simulink model "wbs_sim"  (R2025a)
settings: Solver=FixedStepAuto  StartTime=0.0  StopTime=20  FixedStep=0.001  RelTol=1e-3
undefined symbols (not defined in the file or in its folder): dyaw, L_l, L_r, phi_1l, phi_1r, phi_4l, phi_4r, roll, theta_l, theta_r, x, X, Y, yaw, Z
libraries: sm_lib x86, nesl_utility x28, slpidlib x6
(part 4 of 4)

== system wbs_sim/simscape model/物理系统/左腿/大腿后 ==
  Rigid Transform1 : sm_lib/Frames and Transforms/Rigid Transform  RotationMethod=None  FollAlignAxisA=+X  BaseAlignAxisA=+Y  FollAlignAxisB=+Y  BaseAlignAxisB=+Z  RotationStandardAxis=+Z  RotationAngle=0.0  RotationAngleUnits=deg  RotationArbitraryAxis=[0 0 1]  RotationSequenceAxes=FollowerAxes  RotationSequence=XYX  RotationSequenceAngles=[0 0 0]  RotationSequenceAnglesUnits=deg  RotationMatrix=[1 0 0; 0 1 0; 0 0 1]  Quaternion=[1 0 0 0]  TranslationMethod=StandardAxis  TranslationCartesianOffset=[0 0 0]  TranslationCartesianOffsetUnits=m  TranslationStandardAxis=+X  TranslationStandardOffset=L/2  TranslationStandardOffsetUnits=m  TranslationROffset=0  TranslationROffsetUnits=m  TranslationThetaOffset=0  TranslationThetaOffsetUnits=deg  TranslationZOffset=0  TranslationZOffsetUnits=m
  Rigid Transform3 : sm_lib/Frames and Transforms/Rigid Transform  RotationMethod=None  FollAlignAxisA=+X  BaseAlignAxisA=+Y  FollAlignAxisB=+Y  BaseAlignAxisB=+Z  RotationStandardAxis=+Z  RotationAngle=0.0  RotationAngleUnits=deg  RotationArbitraryAxis=[0 0 1]  RotationSequenceAxes=FollowerAxes  RotationSequence=XYX  RotationSequenceAngles=[0 0 0]  RotationSequenceAnglesUnits=deg  RotationMatrix=[1 0 0; 0 1 0; 0 0 1]  Quaternion=[1 0 0 0]  TranslationMethod=StandardAxis  TranslationCartesianOffset=[0 0 0]  TranslationCartesianOffsetUnits=m  TranslationStandardAxis=+X  TranslationStandardOffset=L/2  TranslationStandardOffsetUnits=m  TranslationROffset=0  TranslationROffsetUnits=m  TranslationThetaOffset=0  TranslationThetaOffsetUnits=deg  TranslationZOffset=0  TranslationZOffsetUnits=m
  Solid : sm_lib/Body Elements/Brick Solid  BrickDimensions=[L H W]  BrickDimensionsUnits=m  ExportEntireGeometry=off  InertiaType=CalculateFromGeometry  BasedOnType=Mass  Density=Mass  DensityUnits=kg/m^3  Mass=mass  MassUnits=kg  CenterOfMass=[0 0 0]  CenterOfMassUnits=m  MomentsOfInertia=[1 1 1]  MomentsOfInertiaUnits=kg*m^2  ProductsOfInertia=[0 0 0]  ProductsOfInertiaUnits=kg*m^2  GraphicType=FromGeometry  MarkerShape=Sphere  MarkerSize=10  GraphicVisPropType=SimpleVisualProperties  GraphicDiffuseColor=[0.6667 0 1]  GraphicOpacity=1.0  GraphicSpecularColor=[0.5 0.5 0.5 1.0]  GraphicAmbientColor=[0.15 0.15 0.15 1.0]  GraphicEmissiveColor=[0.0 0.0 0.0 1.0]  GraphicShininess=75  DoExposeReferenceFrame=on  SerializedFrames=<Frames/>
  Conn1 : PMIOPort  Side=Left
  Conn2 : PMIOPort  Port=2  Side=Right
  connections:
  Solid/RConn1 -- Rigid Transform3/RConn1 -- Rigid Transform1/LConn1
  Conn1/RConn1 -- Rigid Transform3/LConn1
  Rigid Transform1/RConn1 -- Conn2/RConn1

== system wbs_sim/simscape model/物理系统/左腿/小腿前 ==
  Rigid Transform1 : sm_lib/Frames and Transforms/Rigid Transform  RotationMethod=None  FollAlignAxisA=+X  BaseAlignAxisA=+Y  FollAlignAxisB=+Y  BaseAlignAxisB=+Z  RotationStandardAxis=+Z  RotationAngle=0.0  RotationAngleUnits=deg  RotationArbitraryAxis=[0 0 1]  RotationSequenceAxes=FollowerAxes  RotationSequence=XYX  RotationSequenceAngles=[0 0 0]  RotationSequenceAnglesUnits=deg  RotationMatrix=[1 0 0; 0 1 0; 0 0 1]  Quaternion=[1 0 0 0]  TranslationMethod=StandardAxis  TranslationCartesianOffset=[0 0 0]  TranslationCartesianOffsetUnits=m  TranslationStandardAxis=+X  TranslationStandardOffset=L/2  TranslationStandardOffsetUnits=m  TranslationROffset=0  TranslationROffsetUnits=m  TranslationThetaOffset=0  TranslationThetaOffsetUnits=deg  TranslationZOffset=0  TranslationZOffsetUnits=m
  Rigid Transform3 : sm_lib/Frames and Transforms/Rigid Transform  RotationMethod=None  FollAlignAxisA=+X  BaseAlignAxisA=+Y  FollAlignAxisB=+Y  BaseAlignAxisB=+Z  RotationStandardAxis=+Z  RotationAngle=0.0  RotationAngleUnits=deg  RotationArbitraryAxis=[0 0 1]  RotationSequenceAxes=FollowerAxes  RotationSequence=XYX  RotationSequenceAngles=[0 0 0]  RotationSequenceAnglesUnits=deg  RotationMatrix=[1 0 0; 0 1 0; 0 0 1]  Quaternion=[1 0 0 0]  TranslationMethod=StandardAxis  TranslationCartesianOffset=[0 0 0]  TranslationCartesianOffsetUnits=m  TranslationStandardAxis=+X  TranslationStandardOffset=L/2  TranslationStandardOffsetUnits=m  TranslationROffset=0  TranslationROffsetUnits=m  TranslationThetaOffset=0  TranslationThetaOffsetUnits=deg  TranslationZOffset=0  TranslationZOffsetUnits=m
  Solid : sm_lib/Body Elements/Brick Solid  BrickDimensions=[L H W]  BrickDimensionsUnits=m  ExportEntireGeometry=off  InertiaType=CalculateFromGeometry  BasedOnType=Mass  Density=mass  DensityUnits=kg/m^3  Mass=mass  MassUnits=kg  CenterOfMass=[0 0 0]  CenterOfMassUnits=m  MomentsOfInertia=[1 1 1]  MomentsOfInertiaUnits=kg*m^2  ProductsOfInertia=[0 0 0]  ProductsOfInertiaUnits=kg*m^2  GraphicType=FromGeometry  MarkerShape=Sphere  MarkerSize=10  GraphicVisPropType=SimpleVisualProperties  GraphicDiffuseColor=[1 0 1]  GraphicOpacity=1.0  GraphicSpecularColor=[0.5 0.5 0.5 1.0]  GraphicAmbientColor=[0.15 0.15 0.15 1.0]  GraphicEmissiveColor=[0.0 0.0 0.0 1.0]  GraphicShininess=75  DoExposeReferenceFrame=on  SerializedFrames=<Frames/>
  Conn1 : PMIOPort  Side=Left
  Conn2 : PMIOPort  Port=2  Side=Right
  connections:
  Rigid Transform1/RConn1 -- Conn2/RConn1
  Conn1/RConn1 -- Rigid Transform3/LConn1
  Rigid Transform1/LConn1 -- Solid/RConn1 -- Rigid Transform3/RConn1

== system wbs_sim/simscape model/物理系统/左腿/小腿后 ==
  Rigid Transform1 : sm_lib/Frames and Transforms/Rigid Transform  RotationMethod=None  FollAlignAxisA=+X  BaseAlignAxisA=+Y  FollAlignAxisB=+Y  BaseAlignAxisB=+Z  RotationStandardAxis=+Z  RotationAngle=0.0  RotationAngleUnits=deg  RotationArbitraryAxis=[0 0 1]  RotationSequenceAxes=FollowerAxes  RotationSequence=XYX  RotationSequenceAngles=[0 0 0]  RotationSequenceAnglesUnits=deg  RotationMatrix=[1 0 0; 0 1 0; 0 0 1]  Quaternion=[1 0 0 0]  TranslationMethod=StandardAxis  TranslationCartesianOffset=[0 0 0]  TranslationCartesianOffsetUnits=m  TranslationStandardAxis=+X  TranslationStandardOffset=L/2  TranslationStandardOffsetUnits=m  TranslationROffset=0  TranslationROffsetUnits=m  TranslationThetaOffset=0  TranslationThetaOffsetUnits=deg  TranslationZOffset=0  TranslationZOffsetUnits=m
  Rigid Transform3 : sm_lib/Frames and Transforms/Rigid Transform  RotationMethod=None  FollAlignAxisA=+X  BaseAlignAxisA=+Y  FollAlignAxisB=+Y  BaseAlignAxisB=+Z  RotationStandardAxis=+Z  RotationAngle=0.0  RotationAngleUnits=deg  RotationArbitraryAxis=[0 0 1]  RotationSequenceAxes=FollowerAxes  RotationSequence=XYX  RotationSequenceAngles=[0 0 0]  RotationSequenceAnglesUnits=deg  RotationMatrix=[1 0 0; 0 1 0; 0 0 1]  Quaternion=[1 0 0 0]  TranslationMethod=StandardAxis  TranslationCartesianOffset=[0 0 0]  TranslationCartesianOffsetUnits=m  TranslationStandardAxis=+X  TranslationStandardOffset=L/2  TranslationStandardOffsetUnits=m  TranslationROffset=0  TranslationROffsetUnits=m  TranslationThetaOffset=0  TranslationThetaOffsetUnits=deg  TranslationZOffset=0  TranslationZOffsetUnits=m
  Solid : sm_lib/Body Elements/Brick Solid  BrickDimensions=[L H W]  BrickDimensionsUnits=m  ExportEntireGeometry=off  InertiaType=CalculateFromGeometry  BasedOnType=Mass  Density=mass  DensityUnits=kg/m^3  Mass=mass  MassUnits=kg  CenterOfMass=[0 0 0]  CenterOfMassUnits=m  MomentsOfInertia=[1 1 1]  MomentsOfInertiaUnits=kg*m^2  ProductsOfInertia=[0 0 0]  ProductsOfInertiaUnits=kg*m^2  GraphicType=FromGeometry  MarkerShape=Sphere  MarkerSize=10  GraphicVisPropType=SimpleVisualProperties  GraphicDiffuseColor=[1 0 1]  GraphicOpacity=1.0  GraphicSpecularColor=[0.5 0.5 0.5 1.0]  GraphicAmbientColor=[0.15 0.15 0.15 1.0]  GraphicEmissiveColor=[0.0 0.0 0.0 1.0]  GraphicShininess=75  DoExposeReferenceFrame=on  SerializedFrames=<Frames/>
  Conn1 : PMIOPort  Side=Left
  Conn2 : PMIOPort  Port=2  Side=Right
  connections:
  Rigid Transform1/RConn1 -- Conn2/RConn1
  Conn1/RConn1 -- Rigid Transform3/LConn1
  Rigid Transform1/LConn1 -- Solid/RConn1 -- Rigid Transform3/RConn1

== matlab function wbs_sim/controller/left leg transform ==
  data: F input; Tp input; T output; phi1 input; phi4 input
function T = LegTransform(F,Tp,phi1,phi4)
%LegTransform
%    T = LegTransform(F,Tp,PHI1,PHI4)

%    This function was generated by the Symbolic Math Toolbox version 25.1.
%    2025-11-06 00:02:19

t2 = conj(phi1);
t3 = conj(phi4);
t4 = cos(phi1);
t5 = cos(phi4);
t6 = sin(phi1);
t7 = sin(phi4);
t8 = cos(t2);
t9 = cos(t3);
t10 = imag(t4);
t11 = real(t4);
t12 = sin(t2);
t13 = sin(t3);
t14 = imag(t6);
t15 = real(t6);
t16 = t4.*(2.1e+1./1.0e+2);
t17 = t5.*(2.1e+1./1.0e+2);
t18 = t4.*(2.1e+1./2.0e+2);
t19 = t5.*(2.1e+1./2.0e+2);
t20 = t6.*(2.1e+1./1.0e+2);
t21 = t7.*(2.1e+1./1.0e+2);
t22 = t6.*(2.1e+1./2.0e+2);
t23 = t7.*(2.1e+1./2.0e+2);
t24 = -t17;
t25 = -t18;
t26 = -t19;
t27 = -t21;
t28 = -t22;
t29 = -t23;
t30 = t8.*(2.1e+1./1.0e+2);
t31 = t9.*(2.1e+1./1.0e+2);
t32 = t8.*(2.1e+1./2.0e+2);
t33 = t9.*(2.1e+1./2.0e+2);
t34 = t10.*(2.1e+1./1.0e+2);
t35 = t11.*(2.1e+1./1.0e+2);
t36 = t12.*(2.1e+1./1.0e+2);
t37 = t13.*(2.1e+1./1.0e+2);
t38 = t12.*(2.1e+1./2.0e+2);
t39 = t13.*(2.1e+1./2.0e+2);
t40 = t14.*(2.1e+1./1.0e+2);
t41 = t15.*(2.1e+1./1.0e+2);
t42 = -t31;
t43 = -t32;
t44 = -t33;
t45 = -t37;
t46 = -t38;
t47 = -t39;
t48 = -t40;
t49 = t16+t24;
t50 = t18+t26;
t51 = t20+t27;
t52 = t22+t29;
t53 = t49.^2;
t54 = t50.^2;
t55 = t51.^2;
t56 = t52.^2;
t57 = t30+t42;
t58 = t32+t44;
t59 = t36+t45;
t60 = t38+t47;
t63 = t6.*t49.*(2.1e+1./5.0e+1);
t64 = t7.*t49.*(2.1e+1./5.0e+1);
t65 = t4.*t51.*(2.1e+1./5.0e+1);
t66 = t5.*t51.*(2.1e+1./5.0e+1);
t73 = t16.*t52;
t75 = t6.*t50.*(-2.1e+1./1.0e+2);
t76 = t7.*t50.*(-2.1e+1./1.0e+2);
t61 = t59.^2;
t62 = t57.^2;
t67 = -t63;
t68 = -t64;
t71 = -t65;
t72 = -t66;
t77 = t12.*t57.*(2.1e+1./5.0e+1);
t78 = t13.*t57.*(2.1e+1./5.0e+1);
t79 = t8.*t59.*(2.1e+1./5.0e+1);
t80 = t9.*t59.*(2.1e+1./5.0e+1);
t87 = t30.*t60;
t89 = t12.*t58.*(-2.1e+1./1.0e+2);
t90 = t13.*t58.*(-2.1e+1./1.0e+2);
t91 = t53+t55;
t81 = -t77;
t82 = -t78;
t85 = -t79;
t86 = -t80;
t92 = t91.^2;
t93 = t61+t62;
t95 = t63+t71;
t96 = t64+t72;
t97 = t19+t25+t91;
t102 = t22+t65+t67;
t103 = t23+t66+t68;
t94 = -t92;
t98 = t77+t85;
t99 = t78+t86;
t100 = 1.0./t97;
t104 = t33+t43+t93;
t107 = t38+t79+t81;
t108 = t39+t80+t82;
t114 = t91.*t95.*2.0;
t115 = t91.*t96.*2.0;
t101 = t100.^2;
t105 = 1.0./t104;
t109 = t54+t56+t94;
t116 = t93.*t98.*2.0;
t117 = t93.*t99.*2.0;
t122 = t73+t75+t114;
t106 = t105.^2;
t110 = sqrt(t109);
t124 = t87+t89+t116;
t111 = conj(t110);
t112 = 1.0./t110;
t118 = t23+t28+t110;
t113 = 1.0./t111;
t119 = t118.^2;
t120 = t39+t46+t111;
t126 = t100.*t118;
t160 = t101.*t102.*t118;
t161 = t101.*t103.*t118;
t162 = (t112.*t122)./2.0;
t163 = (t112.*(t76+t115+t5.*t52.*(2.1e+1./1.0e+2)))./2.0;
t121 = t120.^2;
t127 = atan(t126);
t129 = t101.*t119;
t164 = -t162;
t165 = -t163;
t166 = t106.*t107.*t120;
t167 = t106.*t108.*t120;
t170 = (t113.*t124)./2.0;
t171 = (t113.*(t90+t117+t9.*t60.*(2.1e+1./1.0e+2)))./2.0;
t128 = conj(t127);
t130 = t127.*2.0;
t131 = t129+1.0;
t151 = t106.*t121;
t168 = t18+t164;
t169 = t19+t165;
t172 = -t170;
t173 = -t171;
t132 = t128.*2.0;
t133 = cos(t130);
t134 = sin(t130);
t141 = 1.0./t131;
t152 = t151+1.0;
t174 = t32+t172;
t175 = t33+t173;
t176 = t100.*t168;
t177 = t100.*t169;
t135 = cos(t132);
t136 = imag(t133);
t137 = real(t133);
t138 = sin(t132);
t139 = imag(t134);
t140 = real(t134);
t142 = t133./4.0;
t143 = t134./4.0;
t153 = 1.0./t152;
t178 = t105.*t174;
t179 = t105.*t175;
t190 = t160+t176;
t191 = t161+t177;
t144 = t135./4.0;
t145 = t136./4.0;
t146 = t137./4.0;
t147 = t138./4.0;
t148 = t139./4.0;
t149 = t140./4.0;
t154 = t16+t142;
t155 = t20+t143;
t192 = t166+t178;
t193 = t167+t179;
t196 = t133.*t141.*t190;
t197 = t133.*t141.*t191;
t198 = t134.*t141.*t190;
t199 = t134.*t141.*t191;
t150 = -t148;
t156 = t155.^2;
t157 = t30+t144;
t158 = t36+t147;
t159 = t154.^2;
t180 = t34+t41+t145+t149;
t181 = t180.^2;
t182 = t156+t159;
t183 = t35+t48+t146+t150;
t184 = t183.^2;
t185 = 1.0./t183;
t187 = sqrt(t182);
t186 = 1.0./t184;
t188 = conj(t187);
t194 = t181+t184;
t189 = 1.0./t188;
t195 = 1.0./t194;
T = [(F.*t189.*(t158.*(t30-(t135.*t153.*t192)./2.0).*2.0-t157.*(t36-(t138.*t153.*t192)./2.0).*2.0))./2.0+Tp.*t184.*t195.*(t185.*(t35+t48+imag(t198)./2.0-real(t196)./2.0)+t180.*t186.*(t34+t41-imag(t196)./2.0-real(t198)./2.0));(F.*t189.*(t135.*t153.*t158.*t193-t138.*t153.*t157.*t193))./2.0-Tp.*t184.*t195.*(t185.*(imag(t199)./2.0-real(t197)./2.0)-t180.*t186.*(imag(t197)./2.0+real(t199)./2.0))];
end

== matlab function wbs_sim/controller/locomotion controller/leg length to K ==
  data: L0 input; K output
function K = L2K(L0)
%L2K
%    K = L2K(L0)

%    This function was generated by the Symbolic Math Toolbox version 25.1.
%    2026-02-26 21:10:48

t2 = L0.^2;
t3 = L0.^3;
mt1 = [L0.*(-8.058054079451216e+1)+t2.*1.111266561106283e+2-t3.*5.570050064105828e+1-1.397100567997982];
mt2 = [L0.*2.226384802799524e+2-t2.*8.445730265674364e+2+t3.*8.571144930355709e+2+2.580676862561292e+1];
mt3 = [L0.*(-3.947395418074744)-t2.*3.005312483744237+t3.*5.586019261862921-8.298781917383621e-2];
mt4 = [L0.*8.790268253518818-t2.*3.342139939748938e+1+t3.*3.050517693395287e+1+3.80632293253745];
mt5 = [L0.*(-2.21995389254811)+t2.*2.521080685468763-t3.*3.567846905058671e-1+2.01840796803208e-2];
mt6 = [L0.*1.124396049178383e-1-t2.*1.801416112273404e+1+t3.*2.325243064366943e+1+2.894654972001914];
mt7 = [L0.*(-4.883517404251372)+t2.*5.109260050214045-t3.*2.378207879607897e-1-1.569855003531288e-2];
mt8 = [L0.*(-5.197957782467425)-t2.*2.565262199021458e+1+t3.*3.788389385141832e+1+7.357148404451421];
mt9 = [L0.*(-7.570604573813285)-t2.*6.547559570516285e+1+t3.*9.081433881099194e+1+1.595196440283853e+1];
mt10 = [L0.*3.492765782807593e+2-t2.*5.115287432331667e+2+t3.*2.364083318770739e+2-1.599625636012706e+1];
mt11 = [L0.*(-5.206067671853355)+t2.*3.482922938476702-t3.*3.21901847650377e-1+2.943195669220958];
mt12 = [L0.*5.2655378179046e+1-t2.*8.229055218753876e+1+t3.*4.521389012376712e+1-4.501773550652623];
K = reshape([mt1,mt2,mt3,mt4,mt5,mt6,mt7,mt8,mt9,mt10,mt11,mt12],2,6);
end

== matlab function wbs_sim/controller/right leg transform ==
  data: F input; Tp input; T output; phi1 input; phi4 input
function T = LegTransform(F,Tp,phi1,phi4)
%LegTransform
%    T = LegTransform(F,Tp,PHI1,PHI4)

%    This function was generated by the Symbolic Math Toolbox version 25.1.
%    2025-11-06 00:02:19

t2 = conj(phi1);
t3 = conj(phi4);
t4 = cos(phi1);
t5 = cos(phi4);
t6 = sin(phi1);
t7 = sin(phi4);
t8 = cos(t2);
t9 = cos(t3);
t10 = imag(t4);
t11 = real(t4);
t12 = sin(t2);
t13 = sin(t3);
t14 = imag(t6);
t15 = real(t6);
t16 = t4.*(2.1e+1./1.0e+2);
t17 = t5.*(2.1e+1./1.0e+2);
t18 = t4.*(2.1e+1./2.0e+2);
t19 = t5.*(2.1e+1./2.0e+2);
t20 = t6.*(2.1e+1./1.0e+2);
t21 = t7.*(2.1e+1./1.0e+2);
t22 = t6.*(2.1e+1./2.0e+2);
t23 = t7.*(2.1e+1./2.0e+2);
t24 = -t17;
t25 = -t18;
t26 = -t19;
t27 = -t21;
t28 = -t22;
t29 = -t23;
t30 = t8.*(2.1e+1./1.0e+2);
t31 = t9.*(2.1e+1./1.0e+2);
t32 = t8.*(2.1e+1./2.0e+2);
t33 = t9.*(2.1e+1./2.0e+2);
t34 = t10.*(2.1e+1./1.0e+2);
t35 = t11.*(2.1e+1./1.0e+2);
t36 = t12.*(2.1e+1./1.0e+2);
t37 = t13.*(2.1e+1./1.0e+2);
t38 = t12.*(2.1e+1./2.0e+2);
t39 = t13.*(2.1e+1./2.0e+2);
t40 = t14.*(2.1e+1./1.0e+2);
t41 = t15.*(2.1e+1./1.0e+2);
t42 = -t31;
t43 = -t32;
t44 = -t33;
t45 = -t37;
t46 = -t38;
t47 = -t39;
t48 = -t40;
t49 = t16+t24;
t50 = t18+t26;
t51 = t20+t27;
t52 = t22+t29;
t53 = t49.^2;
t54 = t50.^2;
t55 = t51.^2;
t56 = t52.^2;
t57 = t30+t42;
t58 = t32+t44;
t59 = t36+t45;
t60 = t38+t47;
t63 = t6.*t49.*(2.1e+1./5.0e+1);
t64 = t7.*t49.*(2.1e+1./5.0e+1);
t65 = t4.*t51.*(2.1e+1./5.0e+1);
t66 = t5.*t51.*(2.1e+1./5.0e+1);
t73 = t16.*t52;
t75 = t6.*t50.*(-2.1e+1./1.0e+2);
t76 = t7.*t50.*(-2.1e+1./1.0e+2);
t61 = t59.^2;
t62 = t57.^2;
t67 = -t63;
t68 = -t64;
t71 = -t65;
t72 = -t66;
t77 = t12.*t57.*(2.1e+1./5.0e+1);
t78 = t13.*t57.*(2.1e+1./5.0e+1);
t79 = t8.*t59.*(2.1e+1./5.0e+1);
t80 = t9.*t59.*(2.1e+1./5.0e+1);
t87 = t30.*t60;
t89 = t12.*t58.*(-2.1e+1./1.0e+2);
t90 = t13.*t58.*(-2.1e+1./1.0e+2);
t91 = t53+t55;
t81 = -t77;
t82 = -t78;
t85 = -t79;
t86 = -t80;
t92 = t91.^2;
t93 = t61+t62;
t95 = t63+t71;
t96 = t64+t72;
t97 = t19+t25+t91;
t102 = t22+t65+t67;
t103 = t23+t66+t68;
t94 = -t92;
t98 = t77+t85;
t99 = t78+t86;
t100 = 1.0./t97;
t104 = t33+t43+t93;
t107 = t38+t79+t81;
t108 = t39+t80+t82;
t114 = t91.*t95.*2.0;
t115 = t91.*t96.*2.0;
t101 = t100.^2;
t105 = 1.0./t104;
t109 = t54+t56+t94;
t116 = t93.*t98.*2.0;
t117 = t93.*t99.*2.0;
t122 = t73+t75+t114;
t106 = t105.^2;
t110 = sqrt(t109);
t124 = t87+t89+t116;
t111 = conj(t110);
t112 = 1.0./t110;
t118 = t23+t28+t110;
t113 = 1.0./t111;
t119 = t118.^2;
t120 = t39+t46+t111;
t126 = t100.*t118;
t160 = t101.*t102.*t118;
t161 = t101.*t103.*t118;
t162 = (t112.*t122)./2.0;
t163 = (t112.*(t76+t115+t5.*t52.*(2.1e+1./1.0e+2)))./2.0;
t121 = t120.^2;
t127 = atan(t126);
t129 = t101.*t119;
t164 = -t162;
t165 = -t163;
t166 = t106.*t107.*t120;
t167 = t106.*t108.*t120;
t170 = (t113.*t124)./2.0;
t171 = (t113.*(t90+t117+t9.*t60.*(2.1e+1./1.0e+2)))./2.0;
t128 = conj(t127);
t130 = t127.*2.0;
t131 = t129+1.0;
t151 = t106.*t121;
t168 = t18+t164;
t169 = t19+t165;
t172 = -t170;
t173 = -t171;
t132 = t128.*2.0;
t133 = cos(t130);
t134 = sin(t130);
t141 = 1.0./t131;
t152 = t151+1.0;
t174 = t32+t172;
t175 = t33+t173;
t176 = t100.*t168;
t177 = t100.*t169;
t135 = cos(t132);
t136 = imag(t133);
t137 = real(t133);
t138 = sin(t132);
t139 = imag(t134);
t140 = real(t134);
t142 = t133./4.0;
t143 = t134./4.0;
t153 = 1.0./t152;
t178 = t105.*t174;
t179 = t105.*t175;
t190 = t160+t176;
t191 = t161+t177;
t144 = t135./4.0;
t145 = t136./4.0;
t146 = t137./4.0;
t147 = t138./4.0;
t148 = t139./4.0;
t149 = t140./4.0;
t154 = t16+t142;
t155 = t20+t143;
t192 = t166+t178;
t193 = t167+t179;
t196 = t133.*t141.*t190;
t197 = t133.*t141.*t191;
t198 = t134.*t141.*t190;
t199 = t134.*t141.*t191;
t150 = -t148;
t156 = t155.^2;
t157 = t30+t144;
t158 = t36+t147;
t159 = t154.^2;
t180 = t34+t41+t145+t149;
t181 = t180.^2;
t182 = t156+t159;
t183 = t35+t48+t146+t150;
t184 = t183.^2;
t185 = 1.0./t183;
t187 = sqrt(t182);
t186 = 1.0./t184;
t188 = conj(t187);
t194 = t181+t184;
t189 = 1.0./t188;
t195 = 1.0./t194;
T = [(F.*t189.*(t158.*(t30-(t135.*t153.*t192)./2.0).*2.0-t157.*(t36-(t138.*t153.*t192)./2.0).*2.0))./2.0+Tp.*t184.*t195.*(t185.*(t35+t48+imag(t198)./2.0-real(t196)./2.0)+t180.*t186.*(t34+t41-imag(t196)./2.0-real(t198)./2.0));(F.*t189.*(t135.*t153.*t158.*t193-t138.*t153.*t157.*t193))./2.0-Tp.*t184.*t195.*(t185.*(imag(t199)./2.0-real(t197)./2.0)-t180.*t186.*(imag(t197)./2.0+real(t199)./2.0))];
end

== matlab function wbs_sim/controller/leg controller/left leg feedforward ==
  data: theta input; feedforward output
function feedforward = FFdf(theta)
%FFdf
%    FEEDFORWARD = FFdf(THETA)

%    This function was generated by the Symbolic Math Toolbox version 25.1.
%    2025-12-06 00:25:32

feedforward = (6.37e+2./1.0e+1)./cos(theta);
end

== matlab function wbs_sim/controller/leg controller/right leg feedforward ==
  data: theta input; feedforward output
function feedforward = FFdf(theta)
%FFdf
%    FEEDFORWARD = FFdf(THETA)

%    This function was generated by the Symbolic Math Toolbox version 25.1.
%    2025-12-06 00:25:32

feedforward = (6.37e+2./1.0e+1)./cos(theta);
end
